simulink model "Simulation_balance_poids_variable_realtime2024"  (R2024a)
settings: Solver=ode4  StartTime=0.0  StopTime=5  FixedStep=step_time  RelTol=1e-3
InitFcn:
  | Initialisation_simulation
  | lookup_table_statespace
values from neighbouring files (symbols this model uses):
  denom_com = [R^2*C^2 3*R*C 1]    [Initialisation_simulation.m]
  denom_cou = [1/(2*pi*165) 1]    [Initialisation_simulation.m]
  denom_pos = [1/(2*pi*80) 1]    [Initialisation_simulation.m]
  dL_table = LUT_Table{:,6}    [Initialisation_simulation.m]
  dPhi_table = LUT_Table{:,7}    [Initialisation_simulation.m]
  gain_com = 0.88    [Initialisation_simulation.m]
  gain_cou = 0.716    [Initialisation_simulation.m]
  gain_mod_cou = Gain_Ampli_Puissance(1)    [Initialisation_simulation.m]
  gain_pos = 1.4925    [Initialisation_simulation.m]
  gain_puis = Gain_Ampli_Puissance(1)    [Initialisation_simulation.m]
  kb_table = LUT_Table{:,5}    [Initialisation_simulation.m]
  kd_pos = -0.207    [Initialisation_simulation.m]
  ki_courant = -325    [Initialisation_simulation.m]
  ki_pos = -27.5    [Initialisation_simulation.m]
  kp_courant = -0.575    [Initialisation_simulation.m]
  kp_pos = 2.325    [Initialisation_simulation.m]
  Lb_table = LUT_Table{:,4}    [Initialisation_simulation.m]
  limVampinf = -511.0    (= -511)    [Initialisation_simulation.m]
  limVampmax = 512.0    (= 512)    [Initialisation_simulation.m]
  nouveaux_coeffs = [0, 0, coeffs_temp]    [Initialisation_simulation.m]
  num_com = 1    [Initialisation_simulation.m]
  num_cou = 1    [Initialisation_simulation.m]
  num_pos = 1    [Initialisation_simulation.m]
  offset_com = -2.5    [Initialisation_simulation.m]
  offset_cou = 3.44    [Initialisation_simulation.m]
  offset_pos = -1.6    [Initialisation_simulation.m]
  per_adc = 1/freq_adc    (= 0.000166666666667)    [Initialisation_simulation.m]
  per_pwm = 1/freq_pwm    (= 6.4e-05)    [Initialisation_simulation.m]
  rb = 1.1745 + 2.349    (= 3.5235)    [Initialisation_simulation.m]
  repos_actionneur = deplacement_statique(idx_force_reduit)    [beam_build_ss.m]    (also in lookup_table_statespace.m = hauteur_encastrement_m + deplacement_statique(idx_force_redu)
  repos_bout = deplacement_statique(idx_bout_reduit)    [beam_build_ss.m]    (also in lookup_table_statespace.m = hauteur_encastrement_m + deplacement_statique(idx_bout_redui)
  sat_com_max = 5    [Initialisation_simulation.m]
  sat_com_min = -5    [Initialisation_simulation.m]
  sat_cou_max = 5    [Initialisation_simulation.m]
  sat_cou_min = 0    [Initialisation_simulation.m]
  sat_pos_max = 5    [Initialisation_simulation.m]
  sat_pos_min = 0    [Initialisation_simulation.m]
  sat_proc_max = 14e-3    (= 0.014)    [Initialisation_simulation.m]    (also in beam_build_ss.m = 1; lookup_table_statespace.m = 1)
  sat_proc_min = 0    [Initialisation_simulation.m]    (also in beam_build_ss.m = -1; lookup_table_statespace.m = -1)
  sat_puis_max = 5    [Initialisation_simulation.m]
  sat_puis_min = -5    [Initialisation_simulation.m]
  SORTIE_POS_MAX = 512.0    (= 512)    [Initialisation_simulation.m]
  SORTIE_POS_MIN = -511.0    (= -511)    [Initialisation_simulation.m]
  step_time = 1/300000    (= 3.33333333333e-06)    [Initialisation_simulation.m]
  Tech = 0.002    [Initialisation_simulation.m]
  Tech_pos = 0.02    [Initialisation_simulation.m]
  tension_selon_distance = polyfit(Distance(1:point_final), Tension(1:point_final), 3)    [Initialisation_simulation.m]
  x_table = LUT_Table{:,2}    [Initialisation_simulation.m]
undefined symbols (not defined in the file or in its folder): etat_boucle_courant, etat_boucle_position, etat_switch_perturbation, etat_switch_pos, etat_switch_vit, etat_test_type, masse_ui, test_pulse_amp, test_pulse_period, test_pulse_width, test_step_time, test_step_val
libraries: simulink_extras x2, simulink x2, cstblocks x1
settings Model: DataTypeOverride=Double  MinMaxOverflowLogging=ForceOff  Creator=johen30  LastModifiedBy=tomur

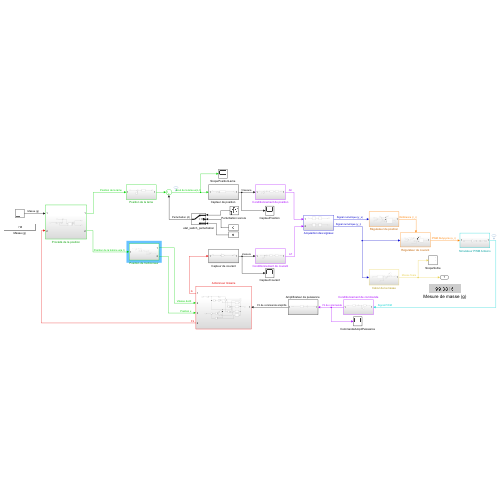
[thumbnail: Simulink's stored preview of the top-level diagram]
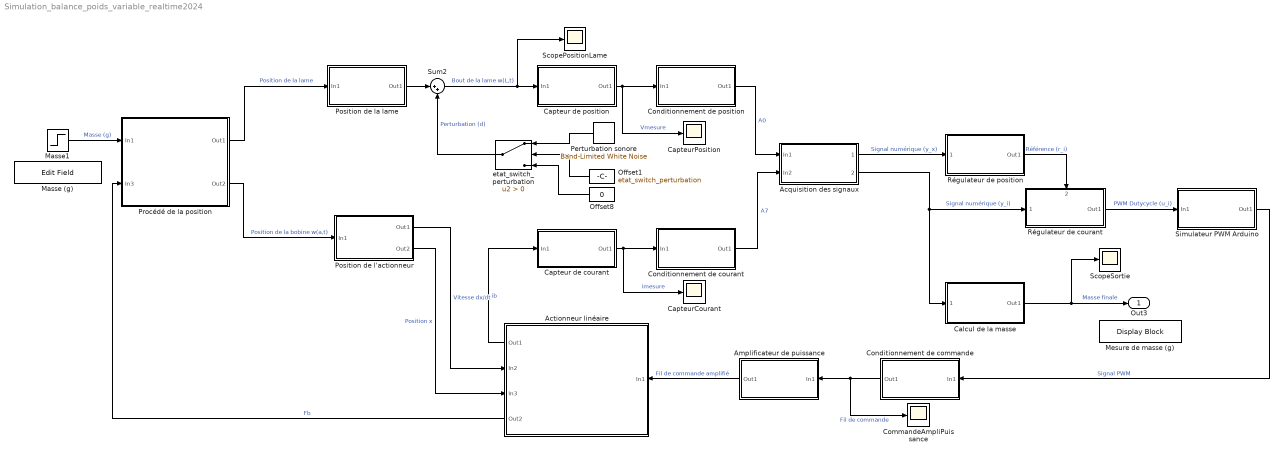
== system Simulation_balance_poids_variable_realtime2024 ==
  Acquisition des signaux : Subsystem
  Actionneur linéaire : Subsystem
      settings: PortSchema="{\"entries\":[{\"content\":{\"sides\":[{\"content\":{\"connectorIds\":[\"In1\"]},\"type\":\"ConnectorPlacement.EquallySpacedRectSide\",\"uuid\":\"16199761-e414-403d-ad97-b0842ee48b95\"},{\"content\":{\"connectorIds\":[\"Out1\",\"In2\",\"In3\",\"Out2\"],\"side\":\"RIGHT\"},\"type\":\"ConnectorPlacement.EquallySpacedRectSide\",\"uuid\":\"eca4d561-471e-4e65-b2d5-07e334f8524a\"},{\"content\":{\"side\":\"TOP\"},\"type\":\"ConnectorPlacement.EquallySpacedRectSide\",\"uuid\":\"5d793a93-245c-48c1-83aa-24e7feb8afb4\"}]},\"type\":\"ConnectorPlacement.EquallySpacedConnector\",\"uuid\":\"f79ebfc1-c7dc-457e-8bf1-e7b29f72d812\"}],\"packageUris\":[\"http://schema.mathworks.com/mf0/Connector/R2020b\"],\"version\":\"1.0\"}"
  "Amplificateur de puissance " : Subsystem
  Calcul de la masse : Subsystem
  Capteur de courant : Subsystem
  "Capteur de position " : Subsystem
  CapteurCourant : Scope
  CapteurPosition : Scope
  CommandeAmpliPuissance : Scope
  Conditionnement de commande : Subsystem
  Conditionnement de courant : Subsystem
  Conditionnement de position : Subsystem
  Masse (g) : EditField  LabelPosition=Hide  ShowInitialText=on  Alignment=Center
  Masse1 : Step  Time=0  After=masse_ui  SampleTime=0
  Mesure de masse (g) : DisplayBlock  LabelPosition=Hide  Transparency=1
  Offset1 : Constant  Value=etat_switch_perturbation
  Offset8 : Constant  Value=0
  "Perturbation sonore " : simulink/Sources/Band-Limited White Noise  Cov=BruitMesure  Ts=0.05  seed=[23341]
  Position de l'actionneur : Subsystem
  Position de la lame : Subsystem
  Procédé de la position : Subsystem
  Régulateur de courant : Subsystem
      settings: PortSchema="{\"entries\":[{\"content\":{\"sides\":[{\"content\":{\"connectorIds\":[\"In1\"]},\"type\":\"ConnectorPlacement.EquallySpacedRectSide\",\"uuid\":\"0c1aee88-c176-4868-9a38-ae31819697f2\"},{\"content\":{\"connectorIds\":[\"Out1\"],\"side\":\"RIGHT\"},\"type\":\"ConnectorPlacement.EquallySpacedRectSide\",\"uuid\":\"955aee84-57a4-48b5-a12a-4136e0ec0ff5\"},{\"content\":{\"connectorIds\":[\"In2\"],\"side\":\"TOP\"},\"type\":\"ConnectorPlacement.EquallySpacedRectSide\",\"uuid\":\"b4792e3f-020f-4e76-ae47-51c6c4b1e10a\"}]},\"type\":\"ConnectorPlacement.EquallySpacedConnector\",\"uuid\":\"cdb56384-e8bf-4241-b5f5-5d2f987823f2\"}],\"packageUris\":[\"http://schema.mathworks.com/mf0/Connector/R2020b\"],\"version\":\"1.0\"}"
  Régulateur de position : Subsystem
  ScopePositionLame : Scope
  ScopeSortie : Scope
  Simulateur PWM Arduino : Subsystem
  Sum2 : Sum  Inputs=|++
  etat_switch_perturbation : Switch  Criteria=u2 > Threshold  SaturateOnIntegerOverflow=off  InputSameDT=off
  Out3 : Outport
  wires:
  "Capteur de position "/1(Out1) -> CapteurPosition/1, Conditionnement de position/1(In1)  "Vmesure"
  Capteur de courant/1(Out1) -> CapteurCourant/1, Conditionnement de courant/1(In1)  "imesure"
  Actionneur linéaire/1(Out1) -> Capteur de courant/1(In1)  "ib"
  "Amplificateur de puissance "/1(Out1) -> Actionneur linéaire/1(In1)  "Fil de commande amplifié"
  Conditionnement de commande/1(Out1) -> "Amplificateur de puissance "/1(In1), CommandeAmpliPuissance/1  "Fil de commande"
  Position de l'actionneur/1(Out1) -> Actionneur linéaire/2(In2)  "Vitesse dx/dt"
  Position de l'actionneur/2(Out2) -> Actionneur linéaire/3(In3)  "Position x"
  Procédé de la position/2(Out2) -> Position de l'actionneur/1(In1)  "Position de la bobine w(a,t)"
  Procédé de la position/1(Out1) -> Position de la lame/1(In1)  "Position de la lame"
  Masse1/1 -> Procédé de la position/1(In1)  "Masse (g)"
  Conditionnement de position/1(Out1) -> Acquisition des signaux/1(In1)  "A0"
  Acquisition des signaux/1(" ") -> Régulateur de position/1(" ")  "Signal numérique (y_x)"
  Conditionnement de courant/1(Out1) -> Acquisition des signaux/2(In2)  "A7"
  Régulateur de position/1(Out1) -> Régulateur de courant/2(" ")  "Référence (r_i)"
  Régulateur de courant/1(Out1) -> Simulateur PWM Arduino/1(In1)  "PWM Dutycycle (u_i)"
  Simulateur PWM Arduino/1(Out1) -> Conditionnement de commande/1(In1)  "Signal PWM"
  Calcul de la masse/1(Out1) -> ScopeSortie/1, Out3/1  "Masse finale"
  Actionneur linéaire/2(Out2) -> Procédé de la position/2(In3)  "Fb"
  Position de la lame/1(Out1) -> Sum2/1
  Sum2/1 -> ScopePositionLame/1, "Capteur de position "/1(In1)  "Bout de la lame w(L,t)"
  Acquisition des signaux/2("  ") -> Calcul de la masse/1("  "), Régulateur de courant/1("  ")  "Signal numérique (y_i)"
  Offset1/1 -> etat_switch_perturbation/2
  etat_switch_perturbation/1 -> Sum2/2  "Perturbation (d)"
  Offset8/1 -> etat_switch_perturbation/3
  "Perturbation sonore "/1 -> etat_switch_perturbation/1

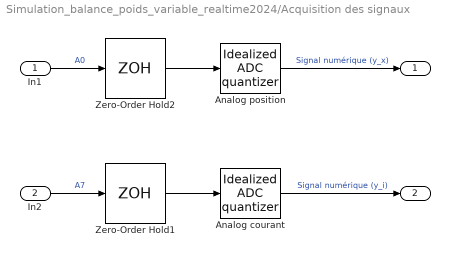
== system Simulation_balance_poids_variable_realtime2024/Acquisition des signaux ==
  In1 : Inport
  In2 : Inport  Port=2
  "Analog courant " : simulink_extras/Additional Discrete/Idealized ADC quantizer  NumberOfConverterBits=res_adc  Vmin=0  Vmax=5  OutputDataType=int16  OutputNegativeValues=off
  Analog position : simulink_extras/Additional Discrete/Idealized ADC quantizer  NumberOfConverterBits=res_adc  Vmin=0  Vmax=5  OutputDataType=int16  OutputNegativeValues=off
  Zero-Order Hold1 : ZeroOrderHold  SampleTime=per_adc
  Zero-Order Hold2 : ZeroOrderHold  SampleTime=per_adc
  " " : Outport
  "  " : Outport  Port=2
  wires:
  Zero-Order Hold2/1 -> Analog position/1
  Analog position/1 -> " "/1  "Signal numérique (y_x)"
  In1/1 -> Zero-Order Hold2/1  "A0"
  Zero-Order Hold1/1 -> "Analog courant "/1
  "Analog courant "/1 -> "  "/1  "Signal numérique (y_i)"
  In2/1 -> Zero-Order Hold1/1  "A7"

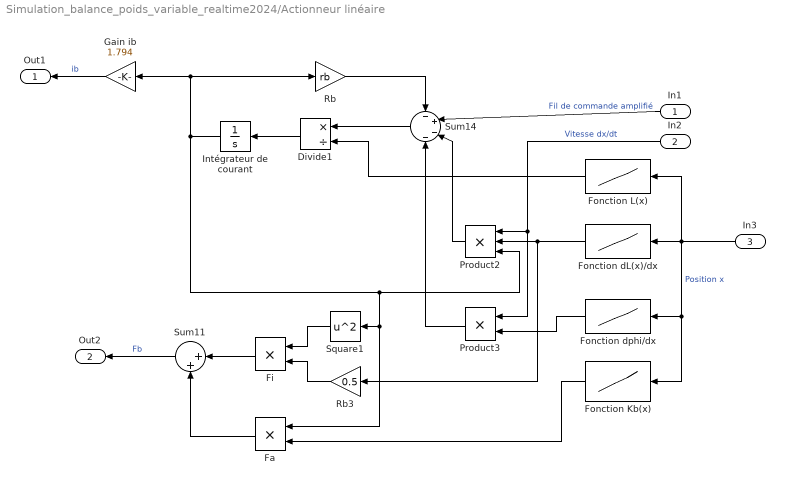
== system Simulation_balance_poids_variable_realtime2024/Actionneur linéaire ==
  In1 : Inport
  In2 : Inport  Port=2
  In3 : Inport  Port=3
  Divide1 : Product  Inputs=*/
  Fa : Product
  Fi : Product
  Fonction Kb(x) : Lookup_n-D  NumberOfTableDimensions=1  BreakpointsForDimension1=x_table  Table=kb_table  InternalRulePriority=Speed  RndMeth=Simplest
  Fonction L(x) : Lookup_n-D  NumberOfTableDimensions=1  BreakpointsForDimension1=x_table  Table=Lb_table  InternalRulePriority=Speed  RndMeth=Simplest
  Fonction dL(x)/dx : Lookup_n-D  NumberOfTableDimensions=1  BreakpointsForDimension1=x_table  Table=dL_table  InternalRulePriority=Speed  RndMeth=Simplest
  Fonction dphi/dx : Lookup_n-D  NumberOfTableDimensions=1  BreakpointsForDimension1=x_table  Table=dPhi_table  InternalRulePriority=Speed  RndMeth=Simplest
  Gain ib : Gain  Gain=1.794
  Intégrateur de courant : Integrator
  Product2 : Product  Inputs=3
  Product3 : Product
  Rb : Gain  Gain=rb
  Rb3 : Gain  Gain=0.5
  Square1 : Math  Operator=square
  Sum11 : Sum  Inputs=|++
  Sum14 : Sum  Inputs=-+--
  Out1 : Outport
  Out2 : Outport  Port=2
  wires:
  In1/1 -> Sum14/2  "Fil de commande amplifié"
  Product2/1 -> Sum14/3
  Fonction dL(x)/dx/1 -> Rb3/1, Product2/2
  Fonction dphi/dx/1 -> Product3/2
  In3/1 -> Fonction dL(x)/dx/1, Fonction L(x)/1, Fonction dphi/dx/1, Fonction Kb(x)/1  "Position x"
  Rb3/1 -> Fi/2
  Square1/1 -> Fi/1
  Fonction Kb(x)/1 -> Fa/2
  In2/1 -> Product2/1, Product3/1  "Vitesse dx/dt"
  Intégrateur de courant/1 -> Rb/1, Gain ib/1, Fa/1, Square1/1, Product2/3
  Product3/1 -> Sum14/4
  Divide1/1 -> Intégrateur de courant/1
  Fi/1 -> Sum11/1
  Fonction L(x)/1 -> Divide1/2
  Fa/1 -> Sum11/2
  Rb/1 -> Sum14/1
  Sum14/1 -> Divide1/1
  Gain ib/1 -> Out1/1  "ib"
  Sum11/1 -> Out2/1  "Fb"

== system Simulation_balance_poids_variable_realtime2024/Amplificateur de puissance  ==
  In1 : Inport
  Gain d'ampli puissance : Gain  Gain=gain_puis
  Saturation puissance : Saturate  UpperLimit=sat_puis_max  LowerLimit=sat_puis_min
  Out1 : Outport
  wires:
  Saturation puissance/1 -> Out1/1  "Fil de commande amplifié"
  Gain d'ampli puissance/1 -> Saturation puissance/1
  In1/1 -> Gain d'ampli puissance/1  "Fil de commande"

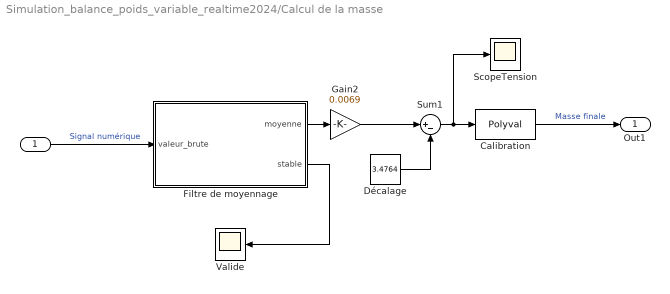
== system Simulation_balance_poids_variable_realtime2024/Calcul de la masse ==
  "  " : Inport
  Calibration : Polyval  Coefs=nouveaux_coeffs
  Décalage : Constant  Value=3.4764
  Filtre de moyennage : MATLAB Function  TreatAsAtomicUnit=on
  Gain2 : Gain  Gain=0.0069
  ScopeTension : Scope
  Sum1 : Sum  Inputs=|+-
  Valide : Scope
  Out1 : Outport
  wires:
  Calibration/1 -> Out1/1  "Masse finale"
  Filtre de moyennage/1(moyenne) -> Gain2/1
  Décalage/1 -> Sum1/2
  Gain2/1 -> Sum1/1
  Sum1/1 -> ScopeTension/1, Calibration/1
  "  "/1 -> Filtre de moyennage/1(valeur_brute)  "Signal numérique"
  Filtre de moyennage/2(stable) -> Valide/1

== system Simulation_balance_poids_variable_realtime2024/Capteur de courant ==
  In1 : Inport
  Gain capteur de courant : Gain  Gain=gain_mod_cou
  Out1 : Outport
  wires:
  Gain capteur de courant/1 -> Out1/1  "imesure"
  In1/1 -> Gain capteur de courant/1  "ib"

== system Simulation_balance_poids_variable_realtime2024/Capteur de position  ==
  In1 : Inport
  Capteur de position : MATLAB Function  TreatAsAtomicUnit=on
  Offset8 : Constant  Value=tension_selon_distance
  Out1 : Outport
  wires:
  Capteur de position/1(tension) -> Out1/1  "Vmesure"
  Offset8/1 -> Capteur de position/2(poly)
  In1/1 -> Capteur de position/1(position)  "Bout de la lame w(L,t)"

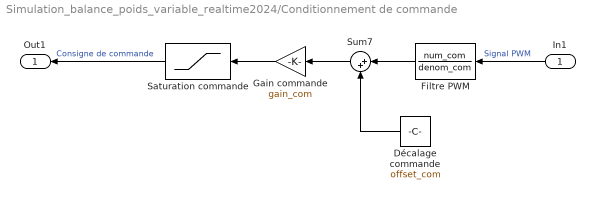
== system Simulation_balance_poids_variable_realtime2024/Conditionnement de commande ==
  In1 : Inport
  Décalage commande : Constant  Value=offset_com
  Filtre PWM : TransferFcn  Numerator=num_com  Denominator=denom_com
  Gain commande : Gain  Gain=gain_com
  Saturation commande : Saturate  UpperLimit=sat_com_max  LowerLimit=sat_com_min
  Sum7 : Sum  Inputs=|++
  Out1 : Outport
  wires:
  Filtre PWM/1 -> Sum7/1
  Décalage commande/1 -> Sum7/2
  Sum7/1 -> Gain commande/1
  Gain commande/1 -> Saturation commande/1
  Saturation commande/1 -> Out1/1  "Consigne de commande"
  In1/1 -> Filtre PWM/1  "Signal PWM"

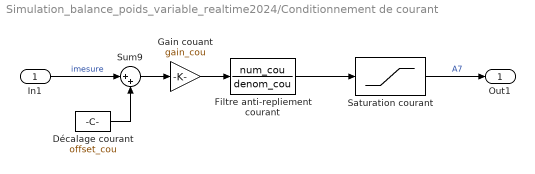
== system Simulation_balance_poids_variable_realtime2024/Conditionnement de courant ==
  In1 : Inport
  Décalage courant : Constant  Value=offset_cou
  Filtre anti-repliement courant : TransferFcn  Numerator=num_cou  Denominator=denom_cou
  Gain couant : Gain  Gain=gain_cou
  Saturation courant : Saturate  UpperLimit=sat_cou_max  LowerLimit=sat_cou_min
  Sum9 : Sum  Inputs=|++
  Out1 : Outport
  wires:
  Saturation courant/1 -> Out1/1  "A7"
  Décalage courant/1 -> Sum9/2
  Gain couant/1 -> Filtre anti-repliement courant/1
  Sum9/1 -> Gain couant/1
  Filtre anti-repliement courant/1 -> Saturation courant/1
  In1/1 -> Sum9/1  "imesure"

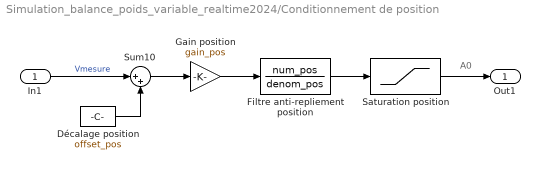
== system Simulation_balance_poids_variable_realtime2024/Conditionnement de position ==
  note: A0
  In1 : Inport
  Décalage position : Constant  Value=offset_pos
  Filtre anti-repliement position : TransferFcn  Numerator=num_pos  Denominator=denom_pos
  Gain position : Gain  Gain=gain_pos
  Saturation position : Saturate  UpperLimit=sat_pos_max  LowerLimit=sat_pos_min  LinearizeAsGain=off
  Sum10 : Sum  Inputs=|++
  Out1 : Outport
  wires:
  Décalage position/1 -> Sum10/2
  Gain position/1 -> Filtre anti-repliement position/1
  Filtre anti-repliement position/1 -> Saturation position/1
  Sum10/1 -> Gain position/1
  In1/1 -> Sum10/1  "Vmesure"
  Saturation position/1 -> Out1/1

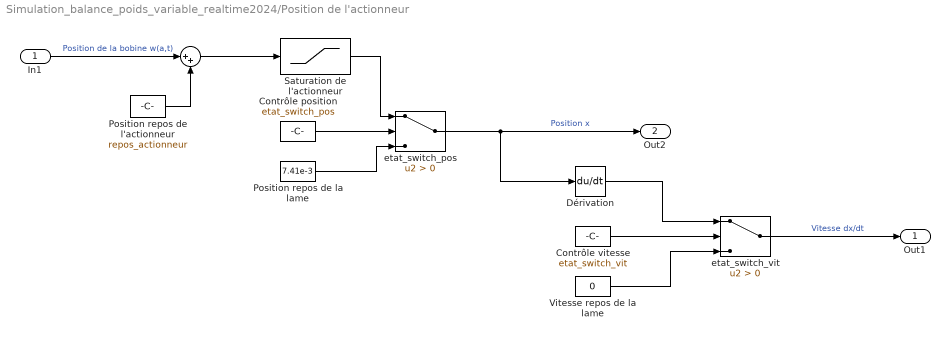
== system Simulation_balance_poids_variable_realtime2024/Position de l'actionneur ==
  In1 : Inport
  "  " : Sum  Inputs=|++
  Contrôle position : Constant  Value=etat_switch_pos
  Contrôle vitesse : Constant  Value=etat_switch_vit
  Dérivation : Derivative
  Position repos de l'actionneur : Constant  Value=repos_actionneur
  Position repos de la lame : Constant  Value=7.41e-3
  Saturation de l'actionneur : Saturate  UpperLimit=sat_proc_max  LowerLimit=sat_proc_min  LinearizeAsGain=off
  Vitesse repos de la lame : Constant  Value=0
  etat_switch_pos : Switch  Criteria=u2 > Threshold  SaturateOnIntegerOverflow=off  InputSameDT=off
  etat_switch_vit : Switch  Criteria=u2 > Threshold  SaturateOnIntegerOverflow=off  InputSameDT=off
  Out1 : Outport
  Out2 : Outport  Port=2
  wires:
  In1/1 -> "  "/1  "Position de la bobine w(a,t)"
  "  "/1 -> Saturation de l'actionneur/1
  Position repos de l'actionneur/1 -> "  "/2
  etat_switch_vit/1 -> Out1/1  "Vitesse dx/dt"
  Dérivation/1 -> etat_switch_vit/1
  Vitesse repos de la lame/1 -> etat_switch_vit/3
  etat_switch_pos/1 -> Dérivation/1, Out2/1  "Position x"
  Position repos de la lame/1 -> etat_switch_pos/3
  Saturation de l'actionneur/1 -> etat_switch_pos/1
  Contrôle position/1 -> etat_switch_pos/2
  Contrôle vitesse/1 -> etat_switch_vit/2

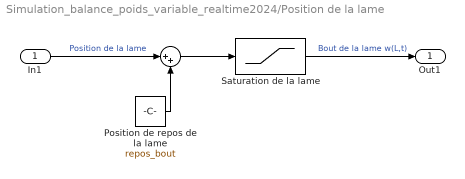
== system Simulation_balance_poids_variable_realtime2024/Position de la lame ==
  In1 : Inport
  "  " : Sum  Inputs=|++
  Position de repos de la lame : Constant  Value=repos_bout
  Saturation de la lame : Saturate  UpperLimit=sat_proc_max  LowerLimit=sat_proc_min  LinearizeAsGain=off
  Out1 : Outport
  wires:
  "  "/1 -> Saturation de la lame/1
  Position de repos de la lame/1 -> "  "/2
  In1/1 -> "  "/1  "Position de la lame"
  Saturation de la lame/1 -> Out1/1  "Bout de la lame w(L,t)"

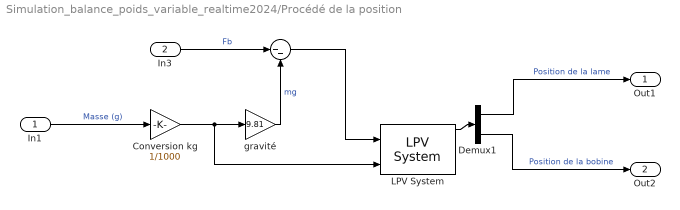
== system Simulation_balance_poids_variable_realtime2024/Procédé de la position ==
  In1 : Inport
  In3 : Inport  Port=2
  "      " : Sum  Inputs=|--
  Conversion kg : Gain  Gain=1/1000
  Demux1 : Demux  Outputs=2
  LPV System : cstblocks/Linear Parameter Varying/LPV System  sys=sys_array  x0=0  opSpecOption=Specify offsets as double arrays  uOffset=0  yOffset=0  xOffset=0  opEquilOption=on  dxOffset=0  sysFixedOption=Use the first model in state-space array  sysFixed=[]  AFixed=false  BFixed=false  CFixed=false  DFixed=false  uDelayFixed=false  yDelayFixed=false  iDelayFixed=false  IMethod=Linear  EMethod=Clip  IndexSearch=Binary search  IndexBegin=on  OutputX=on  OutputXdot=on  OutputLTI=on  OutputOP=on  DataType=double  InitBufferSize=1024  FixedBuffer=off  SimMode=Interpreted execution  Offset=struct
  gravité : Gain  Gain=9.81
  Out1 : Outport
  Out2 : Outport  Port=2
  wires:
  "      "/1 -> LPV System/1
  Demux1/1 -> Out1/1  "Position de la lame"
  gravité/1 -> "      "/2  "mg"
  LPV System/1 -> Demux1/1
  Demux1/2 -> Out2/1  "Position de la bobine"
  In3/1 -> "      "/1  "Fb"
  Conversion kg/1 -> LPV System/2, gravité/1
  In1/1 -> Conversion kg/1  "Masse (g)"

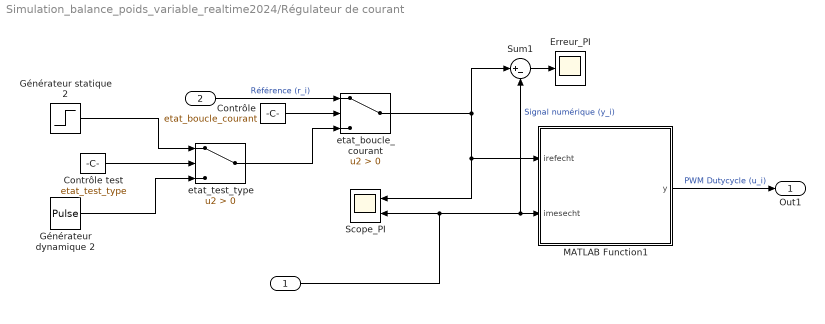
== system Simulation_balance_poids_variable_realtime2024/Régulateur de courant ==
  "  " : Inport
  " " : Inport  Port=2
  Contrôle : Constant  Value=etat_boucle_courant
  Contrôle test : Constant  Value=etat_test_type
  Erreur_PI : Scope
  Générateur dynamique 2 : DiscretePulseGenerator  PulseType=Time based  Amplitude=test_pulse_amp  Period=test_pulse_period  PulseWidth=test_pulse_width
  Générateur statique 2 : Step  Time=test_step_time  After=test_step_val  SampleTime=0
  MATLAB Function1 : MATLAB Function  TreatAsAtomicUnit=on  SystemSampleTime=Tech
  Scope_PI : Scope  NumInputPorts=2
  Sum1 : Sum  Inputs=|+-
  etat_boucle_courant : Switch  Criteria=u2 > Threshold  SaturateOnIntegerOverflow=off  InputSameDT=off
  etat_test_type : Switch  Criteria=u2 > Threshold  SaturateOnIntegerOverflow=off  InputSameDT=off
  Out1 : Outport
  wires:
  etat_boucle_courant/1 -> Sum1/1, Scope_PI/1, MATLAB Function1/1(irefecht)
  MATLAB Function1/1(y) -> Out1/1  "PWM Dutycycle (u_i)"
  " "/1 -> etat_boucle_courant/1  "Référence (r_i)"
  "  "/1 -> Scope_PI/2, Sum1/2, MATLAB Function1/2(imesecht)  "Signal numérique (y_i)"
  etat_test_type/1 -> etat_boucle_courant/3
  Générateur statique 2/1 -> etat_test_type/1
  Générateur dynamique 2/1 -> etat_test_type/3
  Contrôle test/1 -> etat_test_type/2
  Contrôle/1 -> etat_boucle_courant/2
  Sum1/1 -> Erreur_PI/1

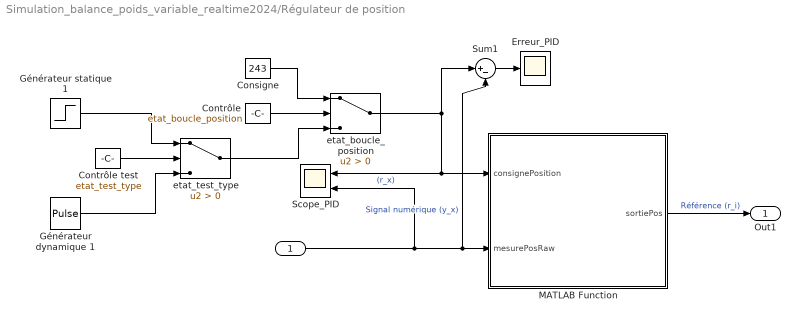
== system Simulation_balance_poids_variable_realtime2024/Régulateur de position ==
  " " : Inport
  Consigne : Constant  Value=243
  Contrôle : Constant  Value=etat_boucle_position
  Contrôle test : Constant  Value=etat_test_type
  Erreur_PID : Scope
  Générateur dynamique 1 : DiscretePulseGenerator  PulseType=Time based  Amplitude=test_pulse_amp  Period=test_pulse_period  PulseWidth=test_pulse_width
  Générateur statique 1 : Step  Time=test_step_time  Before=243  After=test_step_val  SampleTime=0
  MATLAB Function : MATLAB Function  TreatAsAtomicUnit=on  SystemSampleTime=Tech_pos
  Scope_PID : Scope  NumInputPorts=2
  Sum1 : Sum  Inputs=|+-
  etat_boucle_position : Switch  Criteria=u2 > Threshold  SaturateOnIntegerOverflow=off  InputSameDT=off
  etat_test_type : Switch  Criteria=u2 > Threshold  SaturateOnIntegerOverflow=off  InputSameDT=off
  Out1 : Outport
  wires:
  MATLAB Function/1(sortiePos) -> Out1/1  "Référence (r_i)"
  etat_boucle_position/1 -> Sum1/1, Scope_PID/1, MATLAB Function/1(consignePosition)  "(r_x)"
  " "/1 -> MATLAB Function/2(mesurePosRaw), Sum1/2, Scope_PID/2  "Signal numérique (y_x)"
  Générateur statique 1/1 -> etat_test_type/1
  Générateur dynamique 1/1 -> etat_test_type/3
  Consigne/1 -> etat_boucle_position/1
  etat_test_type/1 -> etat_boucle_position/3
  Contrôle/1 -> etat_boucle_position/2
  Contrôle test/1 -> etat_test_type/2
  Sum1/1 -> Erreur_PID/1

== system Simulation_balance_poids_variable_realtime2024/Simulateur PWM Arduino ==
  In1 : Inport
  Ampli pwm : Gain  Gain=5
  PWM contrôle : Gain  Gain=1/1023  OutDataTypeStr=fixdt(1,64, 44)
  PWM1 : simulink/Discontinuities/PWM  DisableCoverage=on  Period=per_pwm  InitialDelay=0  DisallowZeroDutyCycle=off  RunAtFixedTimeIntervals=on  SampleTime=step_time
  Out1 : Outport
  wires:
  PWM contrôle/1 -> PWM1/1
  PWM1/1 -> Ampli pwm/1
  Ampli pwm/1 -> Out1/1
  In1/1 -> PWM contrôle/1  "PWM Dutycycle (u_i)"

== matlab function Simulation_balance_poids_variable_realtime2024/Régulateur de position/MATLAB Function ==
  data: consignePosition input; sortiePos output; mesurePosRaw input; ki_pos parameter; kd_pos parameter; Tech_pos parameter; SORTIE_POS_MIN parameter; SORTIE_POS_MAX parameter; kp_pos parameter
function sortiePos = regulateur_PID_position(consignePosition, mesurePosRaw, ki_pos, kd_pos, Tech_pos, SORTIE_POS_MIN, SORTIE_POS_MAX, kp_pos)
    
    % Constante de temps du filtre dérivé (tirée du code C++ de ton équipe)
    tau_f = 0.09;

    % Calcul des coefficients Tustin à la volée
    den = (2.0 * Tech_pos + 4.0 * tau_f);
    a1 = (4.0 * tau_f) / (Tech_pos + 2.0 * tau_f);
    a2 = (Tech_pos - 2.0 * tau_f) / (Tech_pos + 2.0 * tau_f);

    b0 = (4.0 * kd_pos + ki_pos * Tech_pos^2 + 2.0 * ki_pos * Tech_pos * tau_f + 2.0 * kp_pos * Tech_pos + 4.0 * kp_pos * tau_f) / den;
    b1 = (-8.0 * kd_pos + 2.0 * ki_pos * Tech_pos^2 - 8.0 * kp_pos * tau_f) / den;
    b2 = (4.0 * kd_pos + ki_pos * Tech_pos^2 - 2.0 * ki_pos * Tech_pos * tau_f - 2.0 * kp_pos * Tech_pos + 4.0 * kp_pos * tau_f) / den;

    % Déclaration des variables mémoires (états passés)
    persistent erreurPrecedPos erreurPreced2Pos sortiePrecedPos sortiePreced2Pos;

    % Initialisation au premier appel (t=0)
    if isempty(erreurPrecedPos)
        erreurPrecedPos = 0.0;
        erreurPreced2Pos = 0.0;
        sortiePrecedPos = 0.0;
        sortiePreced2Pos = 0.0;
    end

    % Calcul de l'erreur actuelle
    erreurActuPos = consignePosition - mesurePosRaw;

    % Équation de récurrence (Filtre Tustin)
    sortieBrute = a1 * sortiePrecedPos + ...
                  a2 * sortiePreced2Pos + ...
                  b0 * erreurActuPos + ...
                  b1 * erreurPrecedPos + ...
                  b2 * erreurPreced2Pos;

    % Saturation de la commande de position (Agit aussi comme anti-windup)
    if sortieBrute > SORTIE_POS_MAX
        sortiePos = SORTIE_POS_MAX;
    elseif sortieBrute < SORTIE_POS_MIN
        sortiePos = SORTIE_POS_MIN;
    else
        sortiePos = sortieBrute;
    end

    % Mise à jour des mémoires pour le prochain cycle
    erreurPreced2Pos = erreurPrecedPos;
    erreurPrecedPos  = erreurActuPos;
    sortiePreced2Pos = sortiePrecedPos;
    
    % CRUCIAL : On réinjecte la sortie SATURÉE dans la mémoire
    % C'est ce qui empêche l'intégrale de s'emballer (l'équivalent de l'anti-windup en Tustin)
    sortiePrecedPos  = sortiePos; 

end

== matlab function Simulation_balance_poids_variable_realtime2024/Capteur de position /Capteur de position ==
  data: position input; tension output; poly input
function tension = fct(position, poly)

tension = polyval(poly, position);

== matlab function Simulation_balance_poids_variable_realtime2024/Régulateur de courant/MATLAB Function1 ==
  settings: updateMethod=DISCRETE
  data: irefecht input; y output; imesecht input; kp_courant parameter; ki_courant parameter; Tech parameter; limVampinf parameter; limVampmax parameter
function y = regulateur_PI_courant(irefecht, imesecht, kp_courant, ki_courant, Tech, limVampinf, limVampmax)
    % Calcul de l'erreur interne
    errCur = (irefecht + 512) - imesecht;

    % Création de la mémoire pour l'action intégrale
    persistent intCur;
    if isempty(intCur)
        intCur = 0;
    end

    % 1. Mise à jour de l'intégrale (Euler avant)
    intCur = intCur + (errCur * Tech);

    % 2. Calcul du PI brut
    sortieCurUnsat = (kp_courant * errCur) + (ki_courant * intCur);

    % 3. Saturation de la commande (selon tes limites d'entrée)
    if sortieCurUnsat > limVampmax
        sortieCur = limVampmax;
    elseif sortieCurUnsat < limVampinf
        sortieCur = limVampinf;
    else
        sortieCur = sortieCurUnsat;
    end

    % 4. Anti-windup (Empêche l'intégrale de s'emballer si on sature)
    if ((sortieCurUnsat > limVampmax && errCur > 0.0) || ...
        (sortieCurUnsat < limVampinf && errCur < 0.0))
        intCur = intCur - (errCur * Tech);
    end

    % 5. PWM centré (spécifique au code de ton équipe)
    valeurDutyFloat = 512.0 - sortieCur;

    % 6. Saturation finale du PWM (limites matérielles du timer Arduino : 0 à 1023)
    if valeurDutyFloat > 1023.0
        y = 1023.0;
    elseif valeurDutyFloat < 0.0
        y = 0.0;
    else
        y = valeurDutyFloat;
    end
end

== matlab function Simulation_balance_poids_variable_realtime2024/Calcul de la masse/Filtre de moyennage ==
  data: valeur_brute input; moyenne output; stable output
function [moyenne, stable] = filtre_moyennage(valeur_brute)
    %#codegen
    
    % --- PARAMÈTRES ---
    taille_moyenne = 400;
    taille_fenetre_stable = 20;
    tolerance = 0.75;
    
    % NOUVEAU PARAMÈTRE : Combien de cycles consécutifs pour confirmer la stabilité ?
    % (Ajuste ce chiffre : plus il est grand, plus la LED sera longue à s'allumer, mais plus elle sera fiable)
    cycles_confirmation = 20; 

    % --- VARIABLES MÉMOIRE ---
    persistent buffer_moyenne index_moyenne somme_buffer rempli_moyenne;
    persistent fenetre_stabilite index_stable rempli_stable;
    
    % Nouvelle variable mémoire pour le chronomètre
    persistent compteur_stabilite;

    % Initialisation au tout premier passage de la simulation (t = 0)
    if isempty(buffer_moyenne)
        buffer_moyenne = zeros(taille_moyenne, 1);
        index_moyenne = 1;
        somme_buffer = 0.0;
        rempli_moyenne = false;

        fenetre_stabilite = zeros(taille_fenetre_stable, 1);
        index_stable = 1;
        rempli_stable = false;
        
        compteur_stabilite = 0; % Initialisation du chronomètre
    end

    % =====================================================================
    % 1. CALCUL DE LA MOYENNE GLISSANTE (Circulaire) - INTACT
    % =====================================================================
    ancienne_valeur = buffer_moyenne(index_moyenne);
    somme_buffer = somme_buffer - ancienne_valeur + valeur_brute;
    buffer_moyenne(index_moyenne) = valeur_brute;

    index_moyenne = index_moyenne + 1;
    if index_moyenne > taille_moyenne
        index_moyenne = 1;
        rempli_moyenne = true; 
    end

    if rempli_moyenne
        moyenne = somme_buffer / taille_moyenne;
    else
        nb_elements = index_moyenne - 1;
        if nb_elements == 0
            moyenne = valeur_brute;
        else
            moyenne = somme_buffer / nb_elements;
        end
    end

    % =====================================================================
    % 2. FENÊTRE DE STABILITÉ - INTACT
    % =====================================================================
    fenetre_stabilite(index_stable) = moyenne;

    index_stable = index_stable + 1;
    if index_stable > taille_fenetre_stable
        index_stable = 1;
        rempli_stable = true;
    end

    % =====================================================================
    % 3. ÉVALUATION DE LA STABILITÉ (AVEC ANTI-REBOND)
    % =====================================================================
    if rempli_stable
        ecart = max(fenetre_stabilite) - min(fenetre_stabilite);
        
        % Si on est dans la tolérance, on incrémente le chronomètre
        if ecart <= tolerance
            compteur_stabilite = compteur_stabilite + 1;
        else
            % Si ça sort de la tolérance UNE seule fois, on reset le chronomètre !
            compteur_stabilite = 0; 
        end
        
        % Décision finale pour la LED : a-t-on attendu assez longtemps ?
        if compteur_stabilite >= cycles_confirmation
            stable = 1; 
            compteur_stabilite = cycles_confirmation; % On bloque le compteur pour éviter un "overflow"
        else
            stable = 0; 
        end
    else
        stable = 0; 
    end
end
